simulink model "adaptable_1c_bis"  (Simulink 5.0)
settings: Solver=ode45  StartTime=0.0  StopTime=10.0  RelTol=1e-3
undefined symbols (not defined in the file): A, B, Blockset_Practica2, Diseño
libraries: simulink x6, dsparch4 x2, dspstat3 x2, dspsigops x1
settings Model: LastModifiedBy=pc1

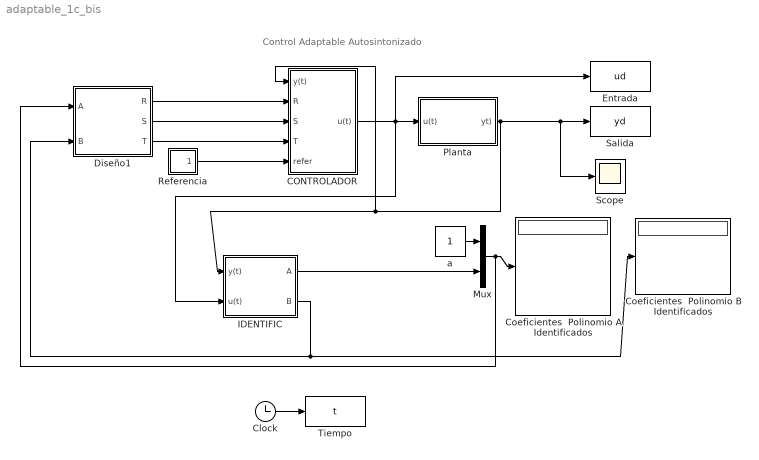
== system adaptable_1c_bis ==
  note: Control Adaptable Autosintonizado
  CONTROLADOR : Subsystem
  Clock : Clock
      settings: Decimation=10
  Coeficientes  Polinomio A Identificados : Display
  Coeficientes  Polinomio B Identificados : Display
  Diseño1 : Subsystem  AncestorBlock=Blockset_Practica2/Diseño  mask{Am=[1 -1.6 .6925 .10475 -.1364 .00242], A0=1}
      mask Display: disp('Diseño')
  Entrada : ToWorkspace  VariableName=ud  SampleTime=.1  SaveFormat=Array
  IDENTIFIC : Subsystem
  Mux : Mux  Inputs=2
  Planta : Subsystem
  Referencia : Subsystem  mask{R=2, A=1}
      mask prompts: R "Seleccion de Referencia"; A "Amplitud de U(t)=Escalon"
  Salida : ToWorkspace  VariableName=yd  SampleTime=.1  SaveFormat=Array
  Scope : Scope
      settings: TimeRange=10  YMin=0  YMax=1.4
  Tiempo : ToWorkspace  VariableName=t  SampleTime=.1  SaveFormat=Array
  a : Constant
  wires:
  Planta/1(yt)) -> Salida/1, Scope/1, CONTROLADOR/1(y(t)), IDENTIFIC/1(y(t))
  Clock/1 -> Tiempo/1
  CONTROLADOR/1(u(t)) -> Entrada/1, Planta/1(u(t)), IDENTIFIC/2(u(t))
  Referencia/1(U(t)) -> CONTROLADOR/5(refer)
  Diseño1/1(R) -> CONTROLADOR/2(R)
  Diseño1/2(S) -> CONTROLADOR/3(S)
  Diseño1/3(T) -> CONTROLADOR/4(T)
  a/1 -> Mux/1
  IDENTIFIC/1(A) -> Mux/2
  Mux/1 -> Coeficientes  Polinomio A Identificados/1, Diseño1/1(A)
  IDENTIFIC/2(B) -> Diseño1/2(B), Coeficientes  Polinomio B Identificados/1

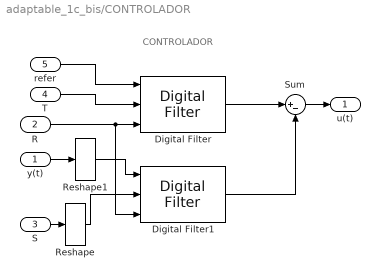
== system adaptable_1c_bis/CONTROLADOR ==
  note: CONTROLADOR
  y(t) : Inport
  R : Inport  Port=2
  S : Inport  Port=3
  T : Inport  Port=4
  refer : Inport  Port=5
  Digital Filter : dsparch4/Digital Filter  TypePopup=IIR (poles & zeros)  IIRFiltStruct=Direct form II  AllPoleFiltStruct=Direct form  FIRFiltStruct=Direct form  CoeffSource=Input port(s)  NumCoeffs=[1 2]  DenCoeffs=[1 0.1]  BiQuadCoeffs=[1 0.3 0.4 1 0.1 0.2]  LatticeCoeffs=[0.2 0.4]  denIgnore=on  FiltPerSampPopup=One filter per frame  IC=0  ICnum=0  ICden=0
  Digital Filter1 : dsparch4/Digital Filter  TypePopup=IIR (poles & zeros)  IIRFiltStruct=Direct form II  AllPoleFiltStruct=Direct form  FIRFiltStruct=Direct form  CoeffSource=Input port(s)  NumCoeffs=[1 2]  DenCoeffs=[1 0.1]  BiQuadCoeffs=[1 0.3 0.4 1 0.1 0.2]  LatticeCoeffs=[0.2 0.4]  denIgnore=on  FiltPerSampPopup=One filter per frame  IC=0  ICnum=0  ICden=0
  Reshape : simulink/Math Operations/Reshape  OutputDimensionality=Column vector  OutputDimensions=[1,1]
  Reshape1 : simulink/Math Operations/Reshape  OutputDimensionality=Column vector  OutputDimensions=[1,1]
  Sum : Sum  Inputs=|+-  SaturateOnIntegerOverflow=on
  u(t) : Outport
  wires:
  Sum/1 -> u(t)/1
  Digital Filter/1 -> Sum/1
  Digital Filter1/1 -> Sum/2
  y(t)/1 -> Reshape1/1
  R/1 -> Digital Filter1/3, Digital Filter/3
  Reshape/1 -> Digital Filter1/2
  T/1 -> Digital Filter/2
  refer/1 -> Digital Filter/1
  S/1 -> Reshape/1
  Reshape1/1 -> Digital Filter1/1

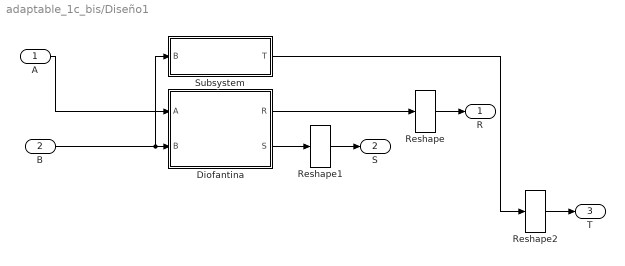
== system adaptable_1c_bis/Diseño1 ==
  A : Inport
  B : Inport  Port=2
  Diofantina : Subsystem  mask{Ac=conv(Am,A0)}
      mask Display: disp('Diofantica')
  Reshape : simulink/Math Operations/Reshape  OutputDimensionality=Column vector  OutputDimensions=[1,1]
  Reshape1 : simulink/Math Operations/Reshape  OutputDimensionality=Column vector  OutputDimensions=[1,1]
  Reshape2 : simulink/Math Operations/Reshape  OutputDimensionality=Column vector  OutputDimensions=[1,1]
  Subsystem : Subsystem  mask{Am=Am, A0=A0}
      mask Display: disp('Polinomio T')
  R : Outport
  S : Outport  Port=2
  T : Outport  Port=3
  wires:
  Subsystem/1(T) -> Reshape2/1
  Diofantina/1(R) -> Reshape/1
  A/1 -> Diofantina/1(A)
  Diofantina/2(S) -> Reshape1/1
  B/1 -> Diofantina/2(B), Subsystem/1(B)
  Reshape/1 -> R/1
  Reshape1/1 -> S/1
  Reshape2/1 -> T/1

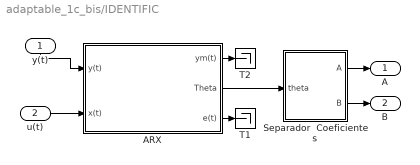
== system adaptable_1c_bis/IDENTIFIC ==
  y(t) : Inport  Orientation=down
  u(t) : Inport  Port=2
  "ARX " : Subsystem  mask{na=3, nb=2, ts=.1, nk=0, L=.995}
      mask prompts: na "na (orden de A)"; nb "nb (orden de B)"; ts "ts (tiempo de muestreo)"; nk "nk (retardo)"; L "lambda (factor de olvido)"
  Separador  Coeficientes : Subsystem  mask{na=3, nb=2}
  T1 : Terminator
  T2 : Terminator
  A : Outport
  B : Outport  Port=2
  wires:
  "ARX "/2(Theta) -> Separador  Coeficientes/1(theta)
  "ARX "/3(e(t)) -> T1/1
  "ARX "/1(ym(t)) -> T2/1
  y(t)/1 -> "ARX "/1(y(t))
  u(t)/1 -> "ARX "/2(x(t))
  Separador  Coeficientes/1(A) -> A/1
  Separador  Coeficientes/2(B) -> B/1

== system adaptable_1c_bis/Planta ==
  u(t) : Inport
  Planta : DiscreteFilter  Numerator=[0 0.53 -0.4]  Denominator=[1 -0.85 0.35 -0.0367]  SampleTime=.1
  yt) : Outport
  wires:
  u(t)/1 -> Planta/1
  Planta/1 -> yt)/1

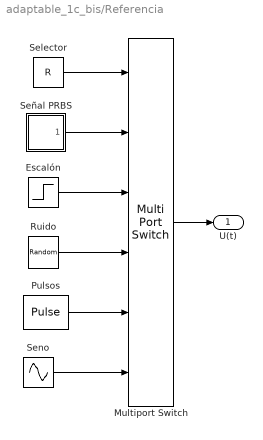
== system adaptable_1c_bis/Referencia ==
  Escalón : Step  Time=.1  After=A  SampleTime=.1
  Multiport Switch : MultiPortSwitch  Inputs=5  SaturateOnIntegerOverflow=on
  Pulsos : DiscretePulseGenerator  PulseType=Time based  PulseWidth=50
  Ruido : UniformRandomNumber  SampleTime=.1
  Selector : Constant  Value=R
  Seno : Sin  Frequency=100  SampleTime=0
  Señal PRBS : Subsystem
  U(t) : Outport
  wires:
  Selector/1 -> Multiport Switch/1
  Señal PRBS/1(u ( t )) -> Multiport Switch/2
  Escalón/1 -> Multiport Switch/3
  Ruido/1 -> Multiport Switch/4
  Multiport Switch/1 -> U(t)/1
  Pulsos/1 -> Multiport Switch/5
  Seno/1 -> Multiport Switch/6

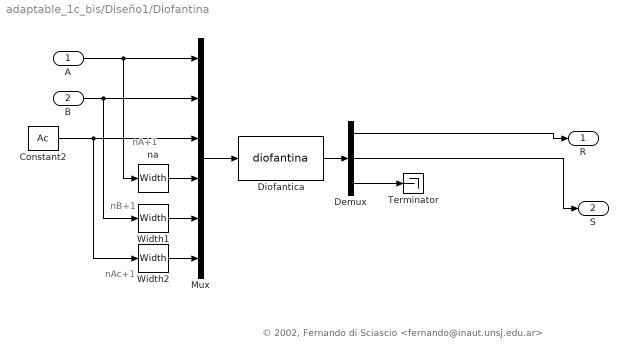
== system adaptable_1c_bis/Diseño1/Diofantina ==
  note: nAc+1
  note: nA+1
  note: nB+1
  note: © 2002, Fernando di Sciascio <fernando@inaut.unsj.edu.ar>
  A : Inport
  B : Inport  Port=2
  Constant2 : Constant  Value=Ac
  Demux : Demux  Outputs="[length(Ac)-length(A)+1  length(A)-1  length(A)+length(B)+length(Ac)-(length(Ac)-length(A)+1)-( length(A)-1 )+3]"
  Diofantica : S-Function  FunctionName=diofantina
      mask Type: S-function: timestwo
      mask Description: Esta S-function resuelve la ecuacion diofantina
      mask Help:
      | Dados los polinomios A, B, Ac y los ordenes de los polinomios R y S esta
      | S-function resuelve la ecuacion diofantina:
      | 
      |     A*R+B*S=Ac
      mask Display: disp('        Diofantina      ');
  Mux : Mux  Inputs=6
  Terminator : Terminator
  Width1 : Width
  Width2 : Width
  na : Width
  R : Outport
  S : Outport  Port=2
  wires:
  Mux/1 -> Diofantica/1
  Constant2/1 -> Mux/3, Width2/1
  Diofantica/1 -> Demux/1
  Demux/3 -> Terminator/1
  A/1 -> Mux/1, na/1
  B/1 -> Mux/2, Width1/1
  Demux/1 -> R/1
  Demux/2 -> S/1
  na/1 -> Mux/4
  Width1/1 -> Mux/5
  Width2/1 -> Mux/6

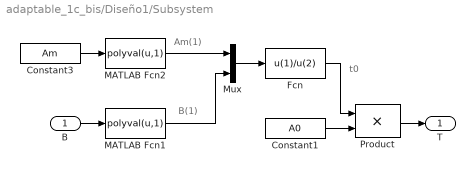
== system adaptable_1c_bis/Diseño1/Subsystem ==
  note: B(1)
  note: Am(1)
  note: t0
  B : Inport
  Constant1 : Constant  Value=A0
  Constant3 : Constant  Value=Am
  Fcn : Fcn  Expr=u(1)/u(2)
  MATLAB Fcn1 : MATLABFcn  MATLABFcn=polyval(u,1)
  MATLAB Fcn2 : MATLABFcn  MATLABFcn=polyval(u,1)
  Mux : Mux  Inputs=2
  Product : Product  SaturateOnIntegerOverflow=on  InputSameDT=on
  T : Outport
  wires:
  Mux/1 -> Fcn/1
  MATLAB Fcn2/1 -> Mux/1
  MATLAB Fcn1/1 -> Mux/2
  Fcn/1 -> Product/1
  Constant3/1 -> MATLAB Fcn2/1
  Product/1 -> T/1
  B/1 -> MATLAB Fcn1/1
  Constant1/1 -> Product/2

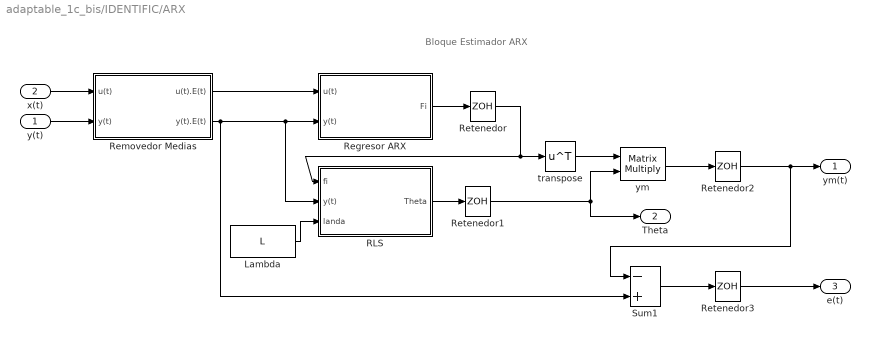
== system adaptable_1c_bis/IDENTIFIC/ARX  ==
  note: Bloque Estimador ARX
  y(t) : Inport
  x(t) : Inport  Port=2
  Lambda : Constant  Value=L  ShowAdditionalParam=on
  RLS : Subsystem
  Regresor ARX : Subsystem
  Removedor Medias : Subsystem
  Retenedor{,1..3} (4 alike) : ZeroOrderHold  SampleTime=ts
  Sum1 : Sum  Inputs=-+  SaturateOnIntegerOverflow=on  InputSameDT=on
  transpose : Math  Operator=transpose
  ym : Product  Multiplication=Matrix(*)  SaturateOnIntegerOverflow=on  InputSameDT=on
  ym(t) : Outport
  Theta : Outport  Port=2
  e(t) : Outport  Port=3
  wires:
  x(t)/1 -> Removedor Medias/1(u(t))
  y(t)/1 -> Removedor Medias/2(y(t))
  Removedor Medias/1(u(t).E(t)) -> Regresor ARX/1(u(t))
  Removedor Medias/2(y(t).E(t)) -> Sum1/2, Regresor ARX/2(y(t)), RLS/2(y(t))
  Regresor ARX/1("Fi ") -> Retenedor/1
  Retenedor/1 -> transpose/1, RLS/1(fi)
  RLS/1(Theta) -> Retenedor1/1
  transpose/1 -> ym/1
  Retenedor1/1 -> ym/2, Theta/1
  ym/1 -> Retenedor2/1
  Retenedor2/1 -> Sum1/1, ym(t)/1
  Sum1/1 -> Retenedor3/1
  Retenedor3/1 -> e(t)/1
  Lambda/1 -> RLS/3(landa)

== system adaptable_1c_bis/IDENTIFIC/Separador  Coeficientes ==
  theta : Inport
  Demux : Demux  Outputs=[na,nb]
  A : Outport
  B : Outport  Port=2
  wires:
  Demux/1 -> A/1
  theta/1 -> Demux/1
  Demux/2 -> B/1

== system adaptable_1c_bis/Referencia/Señal PRBS ==
  Random Number : RandomNumber  Variance=.001  SampleTime=0
  Sign : Signum
  Zero-Order Hold : ZeroOrderHold  SampleTime=.1
  u ( t ) : Outport
  wires:
  Zero-Order Hold/1 -> u ( t )/1
  Sign/1 -> Zero-Order Hold/1
  Random Number/1 -> Sign/1

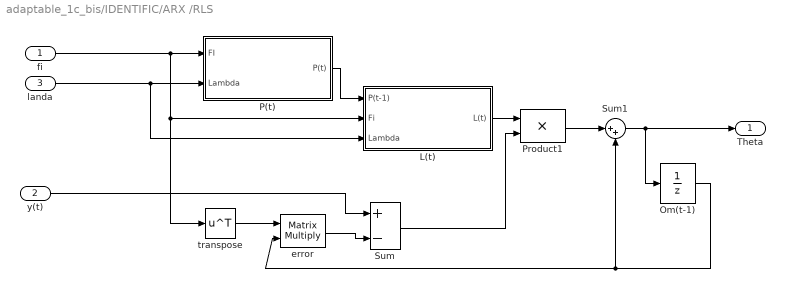
== system adaptable_1c_bis/IDENTIFIC/ARX /RLS ==
  fi : Inport
  y(t) : Inport  Port=2
  landa : Inport  Port=3
  L(t) : Subsystem
  Om(t-1) : UnitDelay  X0="[ -0.8500    0.3500   -0.0367 0.5300   -0.4000]'"  SampleTime=ts
  P(t) : Subsystem
  Product1 : Product  SaturateOnIntegerOverflow=on  InputSameDT=on
  Sum : Sum  Inputs=+-  SaturateOnIntegerOverflow=on  InputSameDT=on
  Sum1 : Sum  Inputs=|++  SaturateOnIntegerOverflow=on  InputSameDT=on
  error : Product  Multiplication=Matrix(*)  SaturateOnIntegerOverflow=on  InputSameDT=on
  transpose : Math  Operator=transpose
  Theta : Outport
  wires:
  transpose/1 -> error/1
  Om(t-1)/1 -> error/2, Sum1/2
  error/1 -> Sum/2
  y(t)/1 -> Sum/1
  Sum/1 -> Product1/2
  Sum1/1 -> Om(t-1)/1, Theta/1
  Product1/1 -> Sum1/1
  L(t)/1(L(t)) -> Product1/1
  P(t)/1("P(t) ") -> L(t)/1(P(t-1))
  fi/1 -> P(t)/1(FI), L(t)/2(Fi), transpose/1
  landa/1 -> P(t)/2(Lambda), L(t)/3(Lambda)

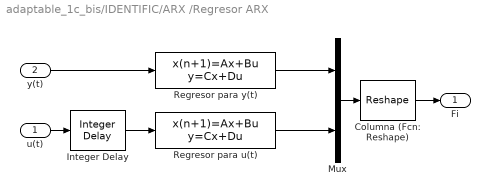
== system adaptable_1c_bis/IDENTIFIC/ARX /Regresor ARX ==
  u(t) : Inport
  y(t) : Inport  Port=2
  "  Columna (Fcn: Reshape)" : simulink/Math Operations/Reshape  OutputDimensionality=Column vector  OutputDimensions=[1,1]
  Integer Delay : dspsigops/Integer Delay  delay=nk  ic=0  reset_popup=None
  Mux : Mux  Inputs=2
  Regresor para u(t) : DiscreteStateSpace  A=[zeros(1,nb);eye(nb-1,nb)]  B=[1,zeros(1,nb-1)]'  C=eye(nb)  D=[zeros(nb,1)]  SampleTime=ts
  Regresor para y(t) : DiscreteStateSpace  A=[zeros(1,na);eye(na-1,na)]  B=[-1,zeros(1,na-1)]'  C=eye(na)  D=[zeros(na,1)]  SampleTime=ts
  "Fi " : Outport
  wires:
  Regresor para y(t)/1 -> Mux/1
  Regresor para u(t)/1 -> Mux/2
  y(t)/1 -> Regresor para y(t)/1
  Mux/1 -> "  Columna (Fcn: Reshape)"/1
  u(t)/1 -> Integer Delay/1
  Integer Delay/1 -> Regresor para u(t)/1
  "  Columna (Fcn: Reshape)"/1 -> "Fi "/1

== system adaptable_1c_bis/IDENTIFIC/ARX /Removedor Medias ==
  u(t) : Inport
  y(t) : Inport  Port=2
  Romovedor de  valores medios : Subsystem
  Romovedor de  valores medios1 : Subsystem
  u(t).E(t) : Outport
  y(t).E(t) : Outport  Port=2
  wires:
  u(t)/1 -> Romovedor de  valores medios/1(x(t))
  Romovedor de  valores medios/1(x(t)-Ex(t)) -> u(t).E(t)/1
  y(t)/1 -> Romovedor de  valores medios1/1(y(t))
  Romovedor de  valores medios1/1(y(t)-Ex(t)) -> y(t).E(t)/1

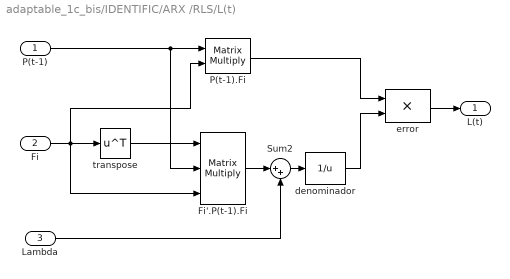
== system adaptable_1c_bis/IDENTIFIC/ARX /RLS/L(t) ==
  P(t-1) : Inport
  Fi : Inport  Port=2
  Lambda : Inport  Port=3
  Fi'.P(t-1).Fi : Product  Inputs=3  Multiplication=Matrix(*)  SaturateOnIntegerOverflow=on  InputSameDT=on
  P(t-1).Fi : Product  Multiplication=Matrix(*)  SaturateOnIntegerOverflow=on  InputSameDT=on
  Sum2 : Sum  Inputs=|++  SaturateOnIntegerOverflow=on  InputSameDT=on
  denominador : Fcn  Expr=1/u
  error : Product  SaturateOnIntegerOverflow=on  InputSameDT=on
  transpose : Math  Operator=transpose
  L(t) : Outport
  wires:
  Fi/1 -> P(t-1).Fi/2, transpose/1, Fi'.P(t-1).Fi/3
  transpose/1 -> Fi'.P(t-1).Fi/1
  Fi'.P(t-1).Fi/1 -> Sum2/1
  Sum2/1 -> denominador/1
  denominador/1 -> error/2
  P(t-1).Fi/1 -> error/1
  P(t-1)/1 -> Fi'.P(t-1).Fi/2, P(t-1).Fi/1
  error/1 -> L(t)/1
  Lambda/1 -> Sum2/2

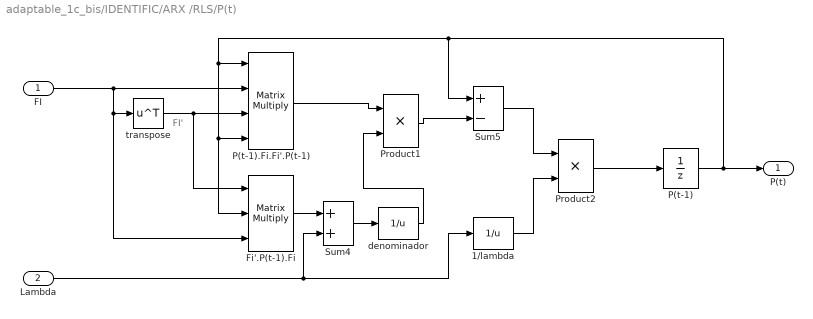
== system adaptable_1c_bis/IDENTIFIC/ARX /RLS/P(t) ==
  note: FI'
  FI : Inport
  Lambda : Inport  Port=2
  1/lambda : Fcn  Expr=1/u
  Fi'.P(t-1).Fi : Product  Inputs=3  Multiplication=Matrix(*)  SaturateOnIntegerOverflow=on  InputSameDT=on
  P(t-1) : UnitDelay  X0=100000*eye(na+nb)  SampleTime=ts
  P(t-1).Fi.Fi'.P(t-1) : Product  Inputs=4  Multiplication=Matrix(*)  SaturateOnIntegerOverflow=on  InputSameDT=on
  Product1 : Product  SaturateOnIntegerOverflow=on  InputSameDT=on
  Product2 : Product  SaturateOnIntegerOverflow=on  InputSameDT=on
  Sum4 : Sum  SaturateOnIntegerOverflow=on  InputSameDT=on
  Sum5 : Sum  Inputs=+-  SaturateOnIntegerOverflow=on  InputSameDT=on
  denominador : Fcn  Expr=1/u
  transpose : Math  Operator=transpose
  "P(t) " : Outport
  wires:
  FI/1 -> Fi'.P(t-1).Fi/3, transpose/1, P(t-1).Fi.Fi'.P(t-1)/2
  transpose/1 -> P(t-1).Fi.Fi'.P(t-1)/3, Fi'.P(t-1).Fi/1
  Lambda/1 -> 1/lambda/1, Sum4/2
  Product2/1 -> P(t-1)/1
  P(t-1)/1 -> Sum5/1, P(t-1).Fi.Fi'.P(t-1)/1, P(t-1).Fi.Fi'.P(t-1)/4, Fi'.P(t-1).Fi/2, "P(t) "/1
  Fi'.P(t-1).Fi/1 -> Sum4/1
  Sum4/1 -> denominador/1
  P(t-1).Fi.Fi'.P(t-1)/1 -> Product1/1
  Product1/1 -> Sum5/2
  Sum5/1 -> Product2/1
  1/lambda/1 -> Product2/2
  denominador/1 -> Product1/2

== system adaptable_1c_bis/IDENTIFIC/ARX /Removedor Medias/Romovedor de  valores medios ==
  x(t) : Inport
  Mean : dspstat3/Mean  run=on  reset_popup=None
  Sum : Sum  Inputs=|-+  SaturateOnIntegerOverflow=on  InputSameDT=on
  Zero-Order Hold : ZeroOrderHold  SampleTime=ts
  x(t)-Ex(t) : Outport
  wires:
  x(t)/1 -> Zero-Order Hold/1
  Zero-Order Hold/1 -> Mean/1, Sum/2
  Mean/1 -> Sum/1
  Sum/1 -> x(t)-Ex(t)/1

== system adaptable_1c_bis/IDENTIFIC/ARX /Removedor Medias/Romovedor de  valores medios1 ==
  y(t) : Inport
  Mean : dspstat3/Mean  run=on  reset_popup=None
  Sum : Sum  Inputs=|-+  SaturateOnIntegerOverflow=on  InputSameDT=on
  Zero-Order Hold : ZeroOrderHold  SampleTime=ts
  y(t)-Ex(t) : Outport
  wires:
  y(t)/1 -> Zero-Order Hold/1
  Zero-Order Hold/1 -> Mean/1, Sum/2
  Mean/1 -> Sum/1
  Sum/1 -> y(t)-Ex(t)/1
